simulink model "Blood_platelet_Count"  (R2022a)
settings: Solver=VariableStepAuto  StartTime=0.0  StopTime=10.0  RelTol=1e-3
libraries: simulink x3
settings Model: Creator=KVJ RAMAN  LastModifiedBy=KVJ RAMAN

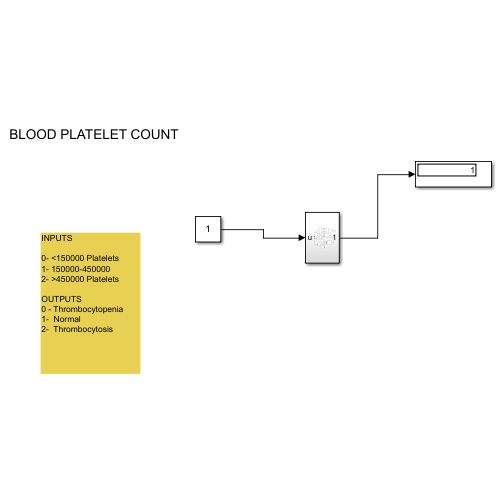
[thumbnail: Simulink's stored preview of the top-level diagram]
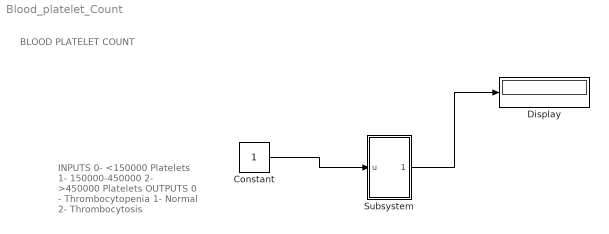
== system Blood_platelet_Count ==
  note: BLOOD PLATELET COUNT
  note: INPUTS
      |
      | 0- <150000 Platelets
      | 1- 150000-450000
      | 2- >450000 Platelets
      |
      | OUTPUTS
      | 0 - Thrombocytopenia
      | 1-  Normal
      | 2-  Thrombocytosis
  Constant : Constant
  Display : Display
  Subsystem : Subsystem
  wires:
  Constant/1 -> Subsystem/1(u)
  Subsystem/1(Out1) -> Display/1

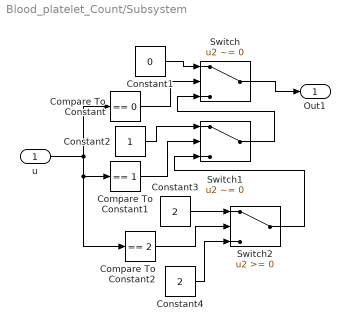
== system Blood_platelet_Count/Subsystem ==
  u : Inport
  Compare To Constant : simulink/Logic and Bit Operations/Compare To Constant  relop===  const=0  OutDataTypeStr=boolean
  Compare To Constant1 : simulink/Logic and Bit Operations/Compare To Constant  relop===  const=1  OutDataTypeStr=boolean
  Compare To Constant2 : simulink/Logic and Bit Operations/Compare To Constant  relop===  const=2  OutDataTypeStr=boolean
  Constant1 : Constant  Value=0
  Constant2 : Constant
  Constant3 : Constant  Value=2
  Constant4 : Constant  Value=2
  Switch : Switch  Criteria=u2 ~= 0  SaturateOnIntegerOverflow=off  InputSameDT=off
  Switch1 : Switch  Criteria=u2 ~= 0  SaturateOnIntegerOverflow=off  InputSameDT=off
  Switch2 : Switch  SaturateOnIntegerOverflow=off  InputSameDT=off
  Out1 : Outport
  wires:
  Switch/1 -> Out1/1
  Constant2/1 -> Switch1/1
  Constant4/1 -> Switch2/3
  Compare To Constant/1 -> Switch/2
  Constant1/1 -> Switch/1
  Compare To Constant2/1 -> Switch2/2
  Compare To Constant1/1 -> Switch1/2
  u/1 -> Compare To Constant/1, Compare To Constant2/1, Compare To Constant1/1
  Switch2/1 -> Switch1/3
  Constant3/1 -> Switch2/1
  Switch1/1 -> Switch/3
